simulink model "MSFartoystyring14"  (R2017b)
settings: Solver=ode45  StartTime=tstart  StopTime=tstop  RelTol=1e-3  EnableMultiTasking=on
values from neighbouring files (symbols this model uses):
  amp = -0.3    [run14.m]    (also in run14_plot.m; run14_ref.m; run_task_1_2.m; run_task_1_4.m)
  c = 1    [run14.m]    (also in run14_plot.m; run14_ref.m; run_task_1_4.m)
  K = x(2)    [run_task_1_2.m]
  Kd = 3*lambda    [run14.m]    (also in run14_ref.m)
  Ki = lambda^3    [run14.m]    (also in run14_ref.m)
  Kp = 3*lambda^2    [run14.m]    (also in run14_ref.m)
  omega_d = 0.008    [run14.m]    (also in run14_plot.m; run14_ref.m; run_task_1_2.m; run_task_1_4.m)
  p0 = zeros(2,1)    [run14.m]    (also in run14_plot.m; run14_ref.m; run_task_1_4.m)
  psi0 = 0    [run14.m]    (also in run14_plot.m; run14_ref.m; run_task_1_4.m)
  r0 = 0    [run14.m]    (also in run14_plot.m; run14_ref.m; run_task_1_4.m)
  T = 1/x(1)    [run_task_1_2.m]
  tsamp = 10    [run14.m]    (also in run14_plot.m; run14_ref.m; run_task_1_4.m)
  v0 = [6.63 0]'    [run14.m]    (also in run14_plot.m; run14_ref.m; run_task_1_4.m)
  w_psi = 0.05    [run14.m]    (also in run14_ref.m)
undefined symbols (not defined in the file or in its folder): msfartoystyring
settings Model: ExtModeAutoUpdateStatusClock=off  Creator=christh  LastModifiedBy=henningward
settings DataIOCC: LimitDataPoints=on  SaveFormat=Array  SignalLoggingSaveFormat=ModelDataLogs
settings OptimizationCC: ExpressionDepthLimit=2147483647  InitFltsAndDblsToZero=on  LifeSpan=inf
settings DebuggingCC: UnderspecifiedInitializationDetection=Classic  MergeDetectMultiDrivingBlocksExec=none  SolverPrmCheckMsg=warning  FcnCallInpInsideContextMsg=warning  StateNameClashWarn=warning  SFUnexpectedBacktrackingDiag=warning  SFNoUnconditionalDefaultTransitionDiag=warning  SFExecutionAtInitializationDiag=none
settings HardwareCC: ProdBitPerPointer=32  ProdBitPerSizeT=32  ProdBitPerPtrDiffT=32  ProdLargestAtomicFloat=None  ProdIntDivRoundTo=Undefined  ProdEndianess=Unspecified  ProdWordSize=32  ProdHWDeviceType=32-bit Generic
settings ModelReferenceCC: PropagateSignalLabelsOutOfModel=off
settings CodeAppCC: StateflowObjectComments=on
settings GRTTargetCC: TargetLangStandard=C89/C90 (ANSI)  GeneratePreprocessorConditionals=Disable all  CombineOutputUpdateFcns=off  GRTInterface=on
settings ConfigComp: CovMetricSettings=dw  CovHtmlReporting=on  CovSaveCumulativeToWorkspaceVar=on  CovSaveSingleToWorkspaceVar=on  CovExternalEMLEnable=off

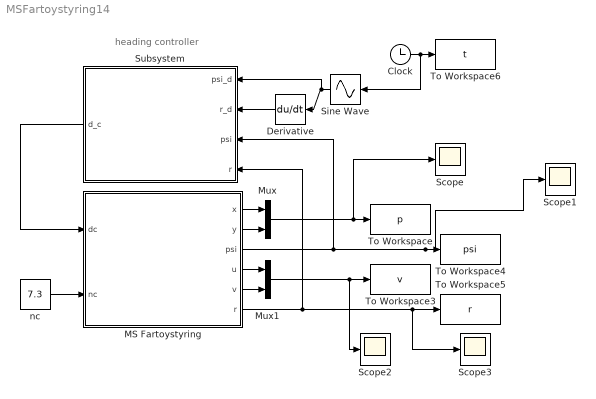
== system MSFartoystyring14 ==
  note: heading controller
  Clock : Clock
  Derivative : Derivative
  MS Fartoystyring : Subsystem  mask(MS Fartoystyring for Assignment 3 G&C){x0=p0(1), y0=p0(2), u0=v0(1), v0=v0(2), psi0=psi0, r0=r0, c=c}
      mask prompts: x0 "x(t0) (m)"; y0 "y(t0) (m)"; u0 "u(t0) (m/s)"; v0 "v(t0) (m/s)"; psi0 "psi(t0) (rad)"; r0 "r(t0) (rad/s)"; c "current (0 or 1)"
      mask help:
      | Block corresponding to Figure 1 in the assignment text. Gives the response of the ship.
      |
      | The design speed of MS Fartoystyring is u=8.23 m/s.
      |
      | Input:
      | dc: commanded rudder (rad), dmax=25*pi/180
      | nc: commanded shaft speed (rad/s), nmax=85*2*pi/60
      |
      | Output:
      | x: north pos (m)
      | y: east pos (m)
      | u: surge (m/s)
      | v: sway (m/s)
      | psi: heading (rad)
      | r: yaw (rad/s)
      mask Help: Comments, bugs and help requests can be directed to the TA. Email on course website.
  Mux : Mux  Inputs=2
  Mux1 : Mux  Inputs=2
  Scope{,1..3} (4 alike) : Scope
  Sine Wave : Sin  TimeSource=Use external signal  Amplitude=amp  Frequency=omega_d  SampleTime=0
  Subsystem : Subsystem
  To Workspace : ToWorkspace  VariableName=p  SampleTime=tsamp
  To Workspace3 : ToWorkspace  VariableName=v  SampleTime=tsamp
  To Workspace4 : ToWorkspace  VariableName=psi  SampleTime=tsamp
  To Workspace5 : ToWorkspace  VariableName=r  SampleTime=tsamp
  To Workspace6 : ToWorkspace  VariableName=t  SampleTime=tsamp
  nc : Constant  Value=7.3
  wires:
  Clock/1 -> Sine Wave/1, To Workspace6/1
  MS Fartoystyring/1(x) -> Mux/1
  MS Fartoystyring/2(y) -> Mux/2
  MS Fartoystyring/4(u) -> Mux1/1
  MS Fartoystyring/5(v) -> Mux1/2
  Mux/1 -> Scope/1, To Workspace/1
  Mux1/1 -> Scope2/1, To Workspace3/1
  MS Fartoystyring/3(psi) -> Subsystem/3("psi "), Scope1/1, To Workspace4/1
  nc/1 -> MS Fartoystyring/2(nc)
  MS Fartoystyring/6(r) -> Subsystem/4(r), Scope3/1, To Workspace5/1
  Subsystem/1("d_c ") -> MS Fartoystyring/1(dc)
  Sine Wave/1 -> Subsystem/1(psi_d), Derivative/1
  Derivative/1 -> Subsystem/2(r_d)

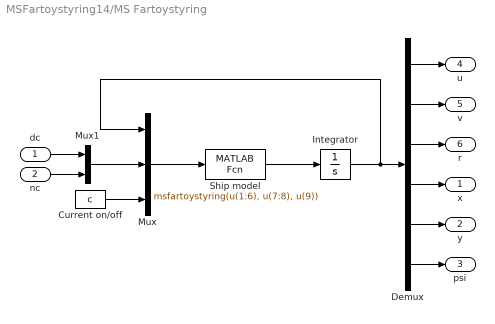
== system MSFartoystyring14/MS Fartoystyring ==
  dc : Inport
  nc : Inport  Port=2
  Current on/off : Constant  Value=c
  Demux : Demux  Outputs=6
  Integrator : Integrator  InitialCondition=[u0 v0 r0 x0 y0 psi0]'
  Mux : Mux  Inputs=3
  Mux1 : Mux  Inputs=2
  Ship model : MATLABFcn  MATLABFcn=msfartoystyring(u(1:6), u(7:8), u(9))  OutputDimensions=6
  x : Outport
  y : Outport  Port=2
  psi : Outport  Port=3
  u : Outport  Port=4
  v : Outport  Port=5
  r : Outport  Port=6
  wires:
  Integrator/1 -> Mux/1, Demux/1
  Mux1/1 -> Mux/2
  dc/1 -> Mux1/1
  nc/1 -> Mux1/2
  Demux/1 -> u/1
  Demux/2 -> v/1
  Demux/3 -> r/1
  Demux/4 -> x/1
  Demux/5 -> y/1
  Demux/6 -> psi/1
  Current on/off/1 -> Mux/3
  Ship model/1 -> Integrator/1
  Mux/1 -> Ship model/1

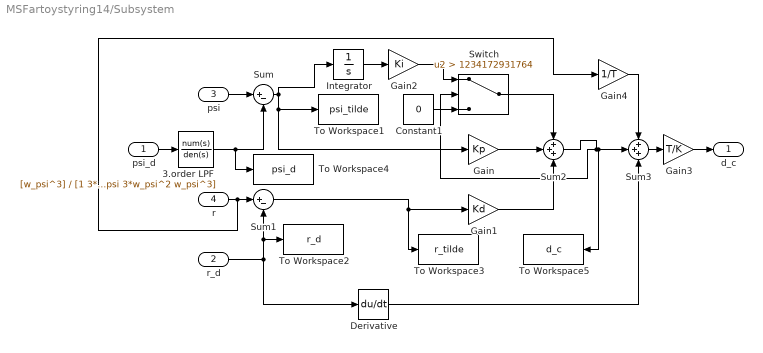
== system MSFartoystyring14/Subsystem ==
  psi_d : Inport
  r_d : Inport  Port=2
  "psi " : Inport  Port=3
  r : Inport  Port=4
  3.order LPF : TransferFcn  Numerator=[w_psi^3]  Denominator=[1 3*w_psi 3*w_psi^2 w_psi^3]
  Constant1 : Constant  Value=0
  Derivative : Derivative
  Gain : Gain  Gain=Kp
  Gain1 : Gain  Gain=Kd
  Gain2 : Gain  Gain=Ki
  Gain3 : Gain  Gain=T/K
  Gain4 : Gain  Gain=1/T
  Integrator : Integrator
  Sum : Sum  Inputs=|+-
  Sum1 : Sum  Inputs=|+-
  Sum2 : Sum  Inputs=+++
  Sum3 : Sum  Inputs=+++
  Switch : Switch  Criteria=u2 > Threshold  Threshold=1234172931764
  To Workspace1 : ToWorkspace  VariableName=psi_tilde  SampleTime=tsamp
  To Workspace2 : ToWorkspace  VariableName=r_d  SampleTime=tsamp
  To Workspace3 : ToWorkspace  VariableName=r_tilde  SampleTime=tsamp
  To Workspace4 : ToWorkspace  VariableName=psi_d  SampleTime=tsamp
  To Workspace5 : ToWorkspace  VariableName=d_c  SampleTime=tsamp
  "d_c " : Outport
  wires:
  r/1 -> Gain4/1, Sum1/1
  "psi "/1 -> Sum/1
  r_d/1 -> Derivative/1, To Workspace2/1, Sum1/2
  Sum1/1 -> To Workspace3/1, Gain1/1
  Integrator/1 -> Gain2/1
  Sum/1 -> Gain/1, To Workspace1/1, Integrator/1
  Gain2/1 -> Switch/1
  Gain/1 -> Sum2/2
  Gain1/1 -> Sum2/3
  psi_d/1 -> 3.order LPF/1
  3.order LPF/1 -> To Workspace4/1, Sum/2
  Constant1/1 -> Switch/3
  Switch/1 -> Sum2/1
  Gain3/1 -> "d_c "/1
  Sum3/1 -> Gain3/1
  Sum2/1 -> Sum3/2, To Workspace5/1, Switch/2
  Derivative/1 -> Sum3/3
  Gain4/1 -> Sum3/1
